simulink model "sim_pemfc"  (R2019a)
settings: Solver=VariableStepAuto  StartTime=0.0  StopTime=2  RelTol=1e-3
libraries: simulink x1
settings Model: Creator=ricardo  LastModifiedBy=ricardo

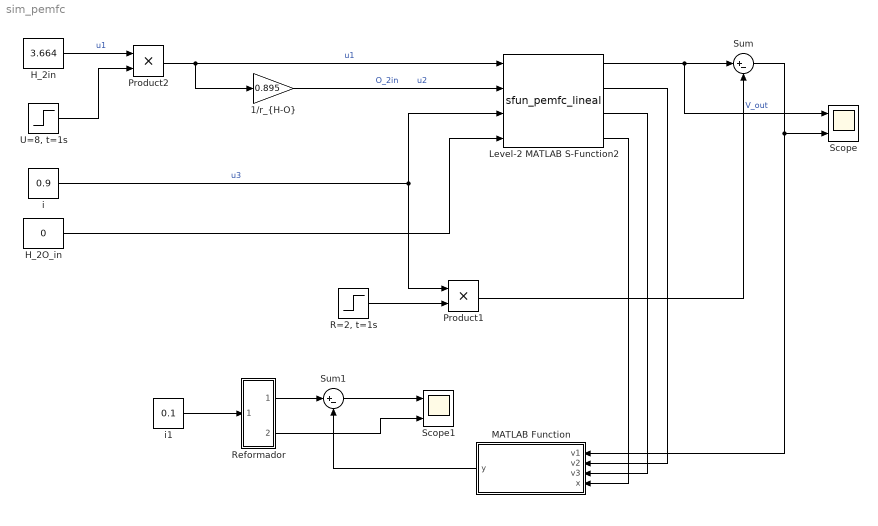
== system sim_pemfc ==
  "1/r_{H-O}" : Gain  Gain=0.895
  H_2O_in : Constant  Value=0
  H_2in : Constant  Value=3.664
  Level-2 MATLAB S-Function2 : M-S-Function  FunctionName=sfun_pemfc_lineal  Parameters=136.7, 6.495, 12.96, 35, 101325, 338.5, 0.6, 0.8, 2, 2, 0.000015, 1.1168, [0, 0, 0, 0, 0]
  MATLAB Function : MATLAB Function  TreatAsAtomicUnit=on
  Product1 : Product
  Product2 : Product
  "R=2, t=1s" : Step  After=2  SampleTime=0
  Reformador : Subsystem
  Scope : Scope  NumInputPorts=2
  Scope1 : Scope  NumInputPorts=2
  Sum : Sum  Inputs=|+-
  Sum1 : Sum  Inputs=|+-
  "U=8, t=1s" : Step  Before=1  After=10  SampleTime=0
  i : Constant  Value=0.9
  i1 : Constant  Value=0.1
  wires:
  H_2O_in/1 -> Level-2 MATLAB S-Function2/4
  Level-2 MATLAB S-Function2/1 -> Scope/1, Sum/1  "V_out"
  "R=2, t=1s"/1 -> Product1/2
  Product1/1 -> Sum/2
  Sum/1 -> Scope/2, MATLAB Function/1(v1)
  H_2in/1 -> Product2/1  "u1"
  Product2/1 -> Level-2 MATLAB S-Function2/1, "1/r_{H-O}"/1  "u1"
  "U=8, t=1s"/1 -> Product2/2
  Level-2 MATLAB S-Function2/2 -> MATLAB Function/2(v2)
  Level-2 MATLAB S-Function2/3 -> MATLAB Function/3(v3)
  Level-2 MATLAB S-Function2/4 -> MATLAB Function/4(x)
  i1/1 -> Reformador/1(u3)
  Reformador/1(H_2) -> Sum1/1
  MATLAB Function/1(y) -> Sum1/2
  "1/r_{H-O}"/1 -> Level-2 MATLAB S-Function2/2  "O_2in       u2"
  i/1 -> Product1/1, Level-2 MATLAB S-Function2/3  "u3"
  Sum1/1 -> Scope1/1
  Reformador/2(O_2) -> Scope1/2

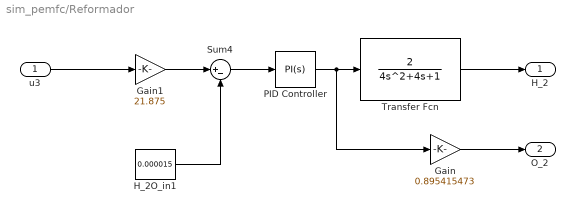
== system sim_pemfc/Reformador ==
  u3 : Inport
  Gain : Gain  Gain=0.895415473
  Gain1 : Gain  Gain=21.875
  H_2O_in1 : Constant  Value=0.000015
  PID Controller : simulink/Continuous/PID Controller  Controller=PI  Form=Parallel  TimeDomain=Continuous-time  SampleTime=-1  IntegratorMethod=Forward Euler  FilterMethod=Forward Euler  ControllerParametersSource=internal  P=2  I=1  D=0  UseFilter=on  N=100  TunerSelectOption=Transfer Function Based (PID Tuner App)  InitialConditionSource=internal  InitialConditionForIntegrator=0  InitialConditionForFilter=0  DifferentiatorICPrevScaledInput=0  ExternalReset=none  TrackingMode=off  Kt=1  LimitOutput=off  UpperSaturationLimit=inf  LowerSaturationLimit=-inf  LinearizeAsGain=on  AntiWindupMode=none  Kb=1  POutMin=[]  POutMax=[]  IOutMin=[]  IOutMax=[]  DOutMin=[]  DOutMax=[]  NOutMin=[]  NOutMax=[]  SumOutMin=[]  SumOutMax=[]  SaturationOutMin=[]  SaturationOutMax=[]  PParamMin=[]  PParamMax=[]  IParamMin=[]  IParamMax=[]  DParamMin=[]  DParamMax=[]  NParamMin=[]  NParamMax=[]  KbParamMin=[]  KbParamMax=[]  KtParamMin=[]  KtParamMax=[]  KbOutMin=[]  KbOutMax=[]  KtOutMin=[]  KtOutMax=[]  IntegratorOutMin=[]  IntegratorOutMax=[]  FilterOutMin=[]  FilterOutMax=[]  SumI1OutMin=[]  SumI1OutMax=[]  SumI2OutMin=[]  SumI2OutMax=[]  SumI3OutMin=[]  SumI3OutMax=[]  SumI4OutMin=[]  SumI4OutMax=[]  SumDOutMin=[]  SumDOutMax=[]  DifferentiatorOutMin=[]  DifferentiatorOutMax=[]  FilterDiffOutCoefMin=[]  FilterDiffOutCoefMax=[]  ReciprocalOutMin=[]  ReciprocalOutMax=[]  SumDenOutMin=[]  SumDenOutMax=[]  SumNumOutMin=[]  SumNumOutMax=[]  DivideOutMin=[]  DivideOutMax=[]  IntegratorContinuousStateAttributes=''  IntegratorStateMustResolveToSignalObject=off  IntegratorRTWStateStorageClass=Auto  FilterContinuousStateAttributes=''  FilterStateMustResolveToSignalObject=off  FilterRTWStateStorageClass=Auto  ParallelPVariant=InternalParameters  IdealPVariant=Disabled  IVariant=InternalParameters  DVariant=Disabled  IntegratorVariant=Continuous  SatVariant=Disabled  AWVariant=Passthrough  PCopyVariant=Disabled  TRVariant=Disabled  FdbkBlocksVariant=Forward  IdealPFdbkVariant=Disabled  SatFdbkVariant=Disabled  DerivativeFilterVariant=Disabled  NVariant=Disabled  NCopyVariant=Disabled_SignalSpec  FilterICVariant=Disabled  IntegratorICVariant=InternalICs  ExternalResetVariant=Disabled  TRSumVariant=Passthrough  SumFdbkVariant=Disabled  SumVariant=Sum_PI
  Sum4 : Sum  Inputs=|+-
  Transfer Fcn : TransferFcn  Numerator=[2]  Denominator=[4 4 1]
  H_2 : Outport
  O_2 : Outport  Port=2
  wires:
  PID Controller/1 -> Gain/1, Transfer Fcn/1
  H_2O_in1/1 -> Sum4/2
  u3/1 -> Gain1/1
  Transfer Fcn/1 -> H_2/1
  Gain/1 -> O_2/1
  Sum4/1 -> PID Controller/1
  Gain1/1 -> Sum4/1

== matlab function sim_pemfc/MATLAB Function ==
  data: v1 input; y output; v2 input; v3 input; x input
function y = nonlinear_control(v1, v2, v3, x)

R = 8.3144; % Constantes de gas ideal
F = 96439; % Constante de Faraday

Ac = 136.7; % Área activa
Va = 6.495; % Volumen del anodo
Vc = 12.96; % Volumen del cátodo
N  = 35; % Número de celdas
Po = 101325; % Presion de operación
T  = 338.5; % Temperatura de operación

K_r = N/(4*F);

NRT = (2*F)/(N*(R^2)*(T^2));

alpha = (Va*x(1)*Po)/(Po-x(1));

beta = (1/(2*Vc))*((1/x(2))-(1/Po))+(1/(Vc*Po));

iota = (2/Va)*((-1/x(1))+(1/Po))+(1/(2*Vc))*((-1/x(2))+(1/Po))-(1/Vc)*((2/x(3))+(1/Po));

u1 = NRT*(alpha*v1-beta*alpha*v2+K_r*Ac*iota*alpha*v3);

y = u1;
